simulink model "ship_extended_model"  (R2022a)
settings: Solver=VariableStepAuto  StartTime=0.0  StopTime=3  RelTol=1e-3
values from neighbouring files (symbols this model uses):
  b = 0.001    [main.m]
  D = 100*[1,0,0 ... (first row only)    [main.m]
  Fb = [0; 0; 2 * roh_water * V_subm * g]    [main.m]
  Fg = [0; 0; -2 * m_boat * g]    [main.m]
  I = I_boat + I_propeller    [main.m]
  k = 0.2    [main.m]
  Ly = 0.206    [main.m]
  Lz = 0.154    [main.m]
  m = m_boat + m_propeller    (= 1.86573735746)    [main.m]
undefined symbols (not defined in the file or in its folder): omega
settings Model: Creator=hhauter  LastModifiedBy=hhauter

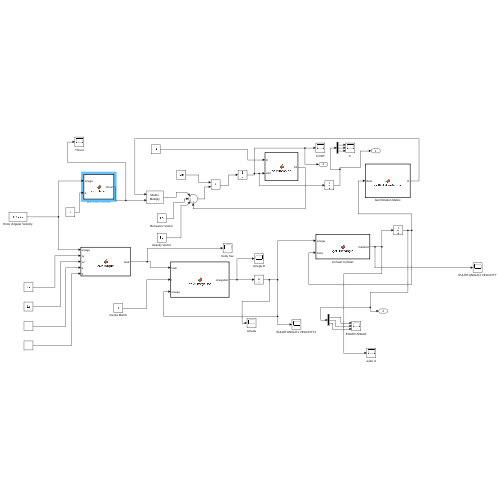
[thumbnail: Simulink's stored preview of the top-level diagram]
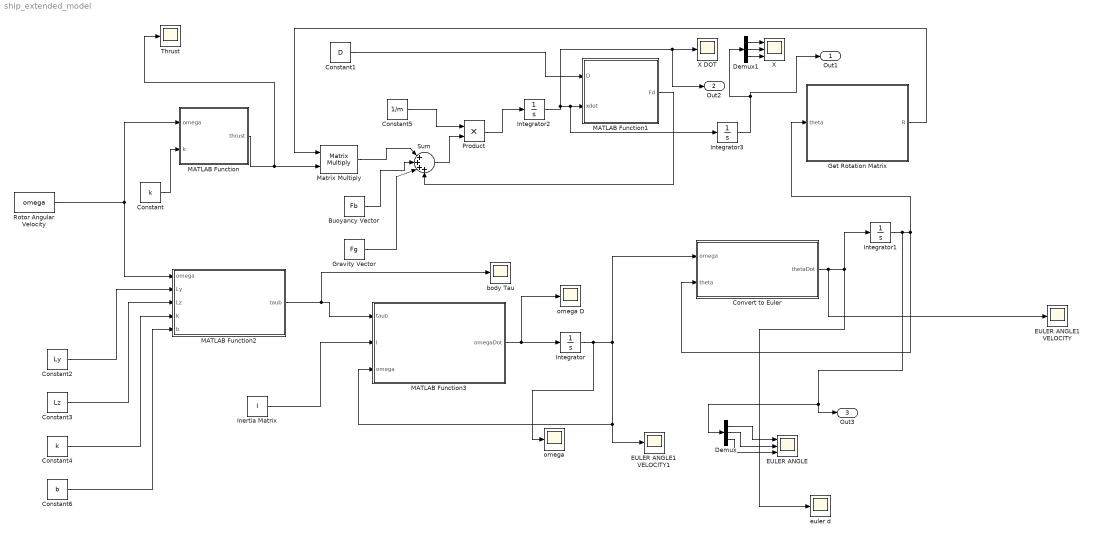
== system ship_extended_model ==
  Buoyancy Vector : Constant  Value=Fb  VectorParams1D=off
  Constant : Constant  Value=k  VectorParams1D=off
  Constant1 : Constant  Value=D  VectorParams1D=off
  Constant2 : Constant  Value=Ly
  Constant3 : Constant  Value=Lz
  Constant4 : Constant  Value=k
  Constant5 : Constant  Value=1/m
  Constant6 : Constant  Value=b
  Convert to Euler : MATLAB Function  TreatAsAtomicUnit=on
  Demux : Demux  Outputs=3
  Demux1 : Demux  Outputs=3
  EULER ANGLE : Scope  NumInputPorts=3
  EULER ANGLE1 VELOCITY : Scope
  EULER ANGLE1 VELOCITY1 : Scope
  Get Rotation Matrix : MATLAB Function  TreatAsAtomicUnit=on
  Gravity Vector : Constant  Value=Fg  VectorParams1D=off
  Inertia Matrix : Constant  Value=I  VectorParams1D=off
  Integrator{,1..3} (4 alike) : Integrator  InitialCondition=[0;0;0]
  MATLAB Function : MATLAB Function  TreatAsAtomicUnit=on
  MATLAB Function1 : MATLAB Function  TreatAsAtomicUnit=on
  MATLAB Function2 : MATLAB Function  TreatAsAtomicUnit=on
  MATLAB Function3 : MATLAB Function  TreatAsAtomicUnit=on
  Matrix Multiply : Product  Multiplication=Matrix(*)
  Product : Product
  Rotor Angular Velocity : Constant  Value=omega  VectorParams1D=off
  Sum : Sum  Inputs=|++++
  Thrust : Scope
  "X " : Scope  NumInputPorts=3
  X DOT : Scope
  body Tau : Scope
  euler d : Scope
  omega : Scope
  omega D : Scope
  Out1 : Outport
  Out2 : Outport  Port=2
  Out3 : Outport  Port=3
  wires:
  Constant/1 -> MATLAB Function/2(k)
  Constant1/1 -> MATLAB Function1/1(D)
  MATLAB Function/1(thrust) -> Thrust/1, Matrix Multiply/2
  Matrix Multiply/1 -> Sum/1
  Gravity Vector/1 -> Sum/3
  MATLAB Function2/1(taub) -> body Tau/1, MATLAB Function3/1(taub)
  Inertia Matrix/1 -> MATLAB Function3/2(I)
  MATLAB Function3/1(omegaDot) -> omega D/1, Integrator/1
  Integrator/1 -> omega/1, Convert to Euler/1(omega), EULER ANGLE1 VELOCITY1/1, MATLAB Function3/3(omega)
  Convert to Euler/1(thetaDot) -> EULER ANGLE1 VELOCITY/1, Integrator1/1, euler d/1
  Integrator1/1 -> Demux/1, Out3/1, Get Rotation Matrix/1(theta), Convert to Euler/2(theta)
  Get Rotation Matrix/1(R) -> Matrix Multiply/1
  Integrator2/1 -> Out2/1, X DOT/1, Integrator3/1, MATLAB Function1/2(xdot)
  Product/1 -> Integrator2/1
  Sum/1 -> Product/2
  Constant5/1 -> Product/1
  Integrator3/1 -> Demux1/1, Out1/1
  Demux/1 -> EULER ANGLE/1
  Demux/2 -> EULER ANGLE/2
  Demux/3 -> EULER ANGLE/3
  Demux1/1 -> "X "/1
  Demux1/2 -> "X "/2
  Demux1/3 -> "X "/3
  Rotor Angular Velocity/1 -> MATLAB Function2/1(omega), MATLAB Function/1(omega)
  Constant2/1 -> MATLAB Function2/2(Ly)
  Constant3/1 -> MATLAB Function2/3(Lz)
  Constant4/1 -> MATLAB Function2/4(k)
  Constant6/1 -> MATLAB Function2/5(b)
  MATLAB Function1/1(Fd) -> Sum/4
  Buoyancy Vector/1 -> Sum/2

== matlab function ship_extended_model/MATLAB Function1 ==
  data: D input; Fd output; xdot input
function Fd = calcDamping(D, xdot)

    Fd = [-D(1,1)*xdot(1); -D(2,2)*xdot(2); -D(3,3)*xdot(3)];

== matlab function ship_extended_model/MATLAB Function ==
  data: omega input; k input; thrust output
function thrust = calcThrust(omega, k)

    thrust = k * [omega(1)^2+omega(2)^2; 0; 0];

== matlab function ship_extended_model/MATLAB Function2 ==
  data: omega input; Ly input; Lz input; taub output; k input; b input
function taub = calcTorque(omega, Ly, Lz, k, b)
taub = [b * (omega(1)^2 - omega(2)^2);
    Lz * k * (- omega(1)^2 - omega(2)^2);
    Ly * k * (omega(1)^2 - omega(2)^2)
    ];

== matlab function ship_extended_model/MATLAB Function3 ==
  data: taub input; omegaDot output; I input; omega input
function omegaDot = calcOmegaDot(taub, I, omega)
    ti = [taub(1) * (1/I(1,1)); 
        taub(2) * (1/I(2,2));
        taub(3) * (1/I(3,3))
        ];
    tw = [( ( I(2,2) - I(3,3) ) /I(1,1) ) * omega(2) * omega(3);
        ( ( I(3,3) - I(1,1) ) / I(2,2) ) * omega(1) * omega(3);
        ( (I(1,1) - I(2,2) ) / I(3,3) ) * omega(1) * omega(2)
        ];
    omegaDot = ti - tw;

== matlab function ship_extended_model/Convert to Euler ==
  data: omega input; thetaDot output; theta input
function thetaDot = getEulerAngle(omega, theta)
    phi = theta(1);
    thetaY = theta(2);
    R = [1, 0 , -sin(thetaY);
        0, cos(phi), cos(thetaY)* sin(phi);
        0, -sin(phi), cos(thetaY) * cos(phi)];
   thetaDot = pinv(R) * omega;

== matlab function ship_extended_model/Get Rotation Matrix ==
  data: theta input; R output
function R = getRotationMatrix(theta)
    omega = theta(1);
    thetay = theta(2);
    phi = theta(3);
    R = [cos(phi)*cos(thetay), cos(phi)*sin(omega)*sin(thetay) - cos(omega)*sin(phi), sin(omega)*sin(phi) + cos(omega)*cos(phi)*sin(thetay); 
        cos(thetay)*sin(phi), cos(omega)*cos(phi) + sin(omega)*sin(phi)*sin(thetay), cos(omega)*sin(phi)*sin(thetay) - cos(phi)*sin(omega); 
        -sin(thetay), cos(thetay)*sin(omega), cos(omega)*cos(thetay)];
%     R = [cos(omega)*cos(thetay), -cos(thetay)*sin(omega), sin(thetay); 
%     cos(phi)*sin(omega) + cos(omega)*sin(phi)*sin(thetay), cos(omega)*cos(phi) - sin(omega)*sin(phi)*sin(thetay), -cos(thetay)*sin(phi); 
%     sin(omega)*sin(phi) - cos(omega)*cos(phi)*sin(thetay), cos(omega)*sin(phi) + cos(phi)*sin(omega)*sin(thetay), cos(phi)*cos(thetay)
%     ];
